simulink model "R_IWPT_mosfet"  (R2022b)
settings: Solver=VariableStepAuto  StartTime=0.0  StopTime=1/100  RelTol=1e-3
libraries: spsDiodeLib x4, spsMosfetLib x4, spsSeriesRLCBranchLib x4, spsVoltageMeasurementLib x3, spsDCVoltageSourceLib x1, spsMutualInductanceLib x1, spspowerguiLib x1
settings Model: Creator=SIDDHARTH  LastModifiedBy=SIDDHARTH

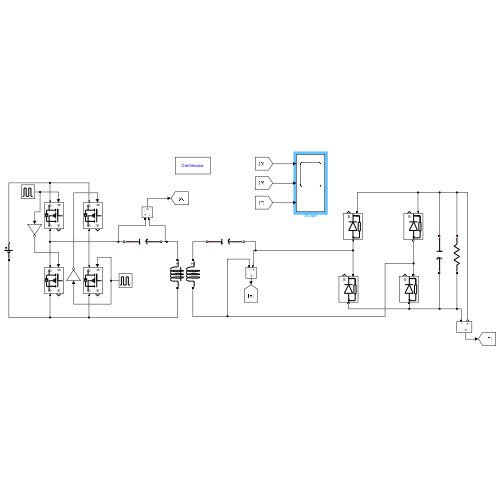
[thumbnail: Simulink's stored preview of the top-level diagram]
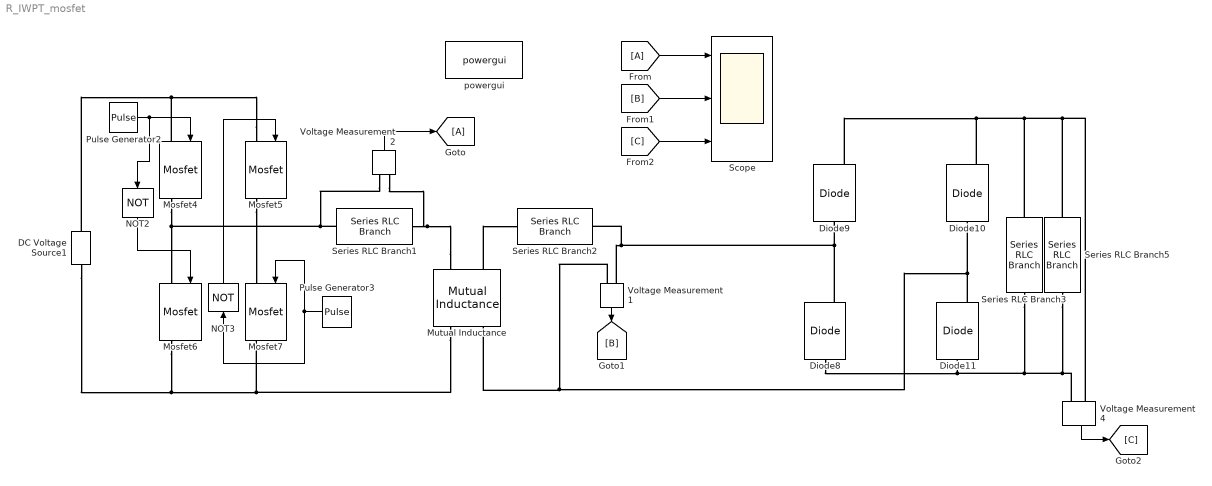
== system R_IWPT_mosfet ==
  DC Voltage Source1 : spsDCVoltageSourceLib/DC Voltage Source  Amplitude=12  Measurements=None
  Diode{8..11} (4 alike) : spsDiodeLib/Diode  Ron=0.001  Lon=0  Vf=0.7  IC=0  UseSnubber=0  Rs=500  Cs=250e-9  Measurements=on
  From : From
  Goto : Goto
  Mosfet{4..7} (4 alike) : spsMosfetLib/Mosfet  Ron=0.1  Lon=0  Rd=0.01  Vfd=0  IC=0  Rs=1e5  Cs=inf  Measurements=on
  Mutual Inductance : spsMutualInductanceLib/Mutual Inductance  LConnTagsString=a|b  RConnTagsString=A|B  TypeOfMutual=Two or three windings with equal mutual terms  NumberOfWindings=3  SelfImpedance1=[1 1/(4*pi*pi*1000*1000*(100e-6))]  SelfImpedance2=[1 1/(4*pi*pi*1000*1000*(100e-6))]  ThreeWindings=off  SelfImpedance3=[ 1.1 1.1e-03]  MutualImpedance=[1.1 0.7838/(4*pi*pi*1000*1000*(100e-6))]  InductanceMatrix="[1.0 0.9  0.9 ;  0.9 1.0  0.9;  0.9 0.9 1.0 ] * 1e-3"  ResistanceMatrix="[1.0 0.9  0.9 ;  0.9 1.0  0.9;  0.9 0.9 1.0 ]"  Measurements=None
      settings: LibrarySourceBlock=sps_lib/Passives/Mutual Inductance
  NOT2 : Logic  Operator=NOT  IconShape=distinctive  AllPortsSameDT=off  OutDataTypeStr=boolean
  NOT3 : Logic  Operator=NOT  IconShape=distinctive  AllPortsSameDT=off  OutDataTypeStr=boolean
  Pulse Generator2 : DiscretePulseGenerator  PulseType=Time based  Period=1/1000  PulseWidth=50
  Pulse Generator3 : DiscretePulseGenerator  PulseType=Time based  Period=1/1000  PulseWidth=50
  Scope : Scope  NumInputPorts=3
  Series RLC Branch1 : spsSeriesRLCBranchLib/Series RLC Branch  LConnTagsString=__new0  RConnTagsString=__new0  BranchType=C  Resistance=1  Inductance=1/(4*pi*pi*(100e-6))  SetiL0=off  InitialCurrent=0  Capacitance=100e-6  Setx0=off  InitialVoltage=0  Measurements=None
  Series RLC Branch2 : spsSeriesRLCBranchLib/Series RLC Branch  LConnTagsString=__new0  RConnTagsString=__new0  BranchType=C  Resistance=1  Inductance=1/(4*pi*pi*(100e-6))  SetiL0=off  InitialCurrent=0  Capacitance=100e-6  Setx0=off  InitialVoltage=0  Measurements=None
  Series RLC Branch3 : spsSeriesRLCBranchLib/Series RLC Branch  LConnTagsString=__new0  RConnTagsString=__new0  BranchType=C  Resistance=1  Inductance=1e-3  SetiL0=off  InitialCurrent=0  Capacitance=100e-6  Setx0=off  InitialVoltage=0  Measurements=None
  Series RLC Branch5 : spsSeriesRLCBranchLib/Series RLC Branch  LConnTagsString=__new0  RConnTagsString=__new0  BranchType=R  Resistance=1000  Inductance=1e-3  SetiL0=off  InitialCurrent=0  Capacitance=1e-6  Setx0=off  InitialVoltage=0  Measurements=None
  Voltage Measurement1 : spsVoltageMeasurementLib/Voltage Measurement  PhasorSimulation=off  OutputType=Complex  PSBequivalent=0
  Voltage Measurement2 : spsVoltageMeasurementLib/Voltage Measurement  PhasorSimulation=off  OutputType=Complex  PSBequivalent=0
  Voltage Measurement4 : spsVoltageMeasurementLib/Voltage Measurement  PhasorSimulation=off  OutputType=Complex  PSBequivalent=0
  powergui : spspowerguiLib/powergui  Priority=1  SimulationMode=Continuous  SampleTime=50e-6  frequency=60  Iterations=50  frequencyindice=0  Pbase=100e6  ErrMax=1e-4  UnitsV=kV  UnitsW=MW  buscounter=0  FunctionMessages=off  echomessages=off  EnableUseOfTLC=off  CurrentSourceSwitches=off  DisableSnubberDevices=off  DisableRonSwitches=off  DisableVfSwitches=off  DisplayEquations=off  AutomaticDiscreteSolvers=off  SolverType=Tustin/Backward Euler (TBE)  Interpol=off  ExternalGateDelay=off  methode=off  Ts=100  x0status=blocks  SPID=on  SwTol=0  HookPort=off  NonlinearTolerance=1e-4  nMaxIteration=100  ContinueOnMaxIteration=off  RestoreLinks=warning  ResistiveCurrentMeasurement=off  Frange=[0:2:500]  Ylog=off  Xlog=on  ShowGrid=off  save=off  variable=ZData  structure=0  ZoomFFT=off  StartTime=0.0  cycles=1  DisplayStyle=1  fundamental=60  FreqAxis=off  MaxFrequency=1000  frequencyindicesteady=1  RmsSteady=1  display=off
  wires:
  Voltage Measurement4/1 -> [C]
  Voltage Measurement1/1 -> [B]
  NOT2/1 -> Mosfet6/1
  Voltage Measurement2/1 -> Goto/1
  NOT3/1 -> Mosfet5/1
  Pulse Generator3/1 -> Mosfet7/1, NOT3/1
  Pulse Generator2/1 -> NOT2/1, Mosfet4/1
  From/1 -> Scope/1
  [B] -> Scope/2
  [C] -> Scope/3
  connections:
  Diode11/LConn1 -- Diode8/LConn1 -- Series RLC Branch3/RConn1 -- Series RLC Branch5/RConn1 -- Voltage Measurement4/LConn2
  Mosfet7/RConn1 -- Mutual Inductance/RConn1 -- DC Voltage Source1/LConn1 -- Mosfet6/RConn1
  Mutual Inductance/RConn2 -- Voltage Measurement1/LConn2 -- Diode10/LConn1 -- Diode11/RConn1
  Mosfet5/LConn1 -- DC Voltage Source1/RConn1 -- Mosfet4/LConn1
  Voltage Measurement4/LConn1 -- Series RLC Branch5/LConn1 -- Diode9/RConn1 -- Diode10/RConn1 -- Series RLC Branch3/LConn1
  Mutual Inductance/LConn1 -- Series RLC Branch1/RConn1 -- Voltage Measurement2/LConn2
  Series RLC Branch1/LConn1 -- Mosfet4/RConn1 -- Mosfet6/LConn1 -- Voltage Measurement2/LConn1
  Series RLC Branch2/RConn1 -- Diode8/RConn1 -- Diode9/LConn1 -- Voltage Measurement1/LConn1
  Mutual Inductance/LConn2 -- Series RLC Branch2/LConn1
  Mosfet5/RConn1 -- Mosfet7/LConn1
